simulink model "modelo_naolinear"  (R2018a)
settings: Solver=ode4  StartTime=0.0  StopTime=T_sim  FixedStep=dt  RelTol=1e-3  EnableMultiTasking=on
InitFcn:
  | modelo_naolinear_params
values from neighbouring files (symbols this model uses):
  B22 = B(7:12,2:4)    [main_model2.m]    (also in main_modelo_linear_v1.m; main_modelo_nao_linear_v2.m; modelo_naolinear.m; modelo_naolinear_params.m)
  feed_forward_motor = 2.0    (= 2)    [modelo_naolinear.m]    (also in modelo_naolinear_params.m = 0.5)
  G = inv(K*B22*inv(R)*B22'-A22')*C'*Q    [modelo_naolinear.m]    (also in modelo_naolinear_params.m)
  g = 9.8    [main_model1.m]    (also in main_model2.m; main_modelo_linear_v1.m; main_modelo_linear_v2.m; main_modelo_nao_linear_v1.m)
  incluir_din_motor = -1    [main_model1.m]    (also in main_model2.m; main_modelo_nao_linear_v1.m = 1; main_modelo_nao_linear_v2.m; modelo_naolinear.m = 1)
  Ir = 1e-3    (= 0.001)    [main_model1.m]    (also in main_model2.m; main_modelo_linear_v1.m = 0.01; main_modelo_linear_v2.m = 0.01; main_modelo_nao_linear_v1.m)
  Ixx = 1e-2    (= 0.01)    [main_model1.m]    (also in main_model2.m; main_modelo_linear_v1.m; main_modelo_linear_v2.m; main_modelo_nao_linear_v1.m)
  Iyy = 1e-2    (= 0.01)    [main_model1.m]    (also in main_model2.m; main_modelo_linear_v1.m; main_modelo_linear_v2.m; main_modelo_nao_linear_v1.m)
  Izz = 1.8e-2    (= 0.018)    [main_model1.m]    (also in main_model2.m; main_modelo_linear_v1.m; main_modelo_linear_v2.m; main_modelo_nao_linear_v1.m)
  K = are(A22, B22*inv(R)*B22',C'*Q*C)    [modelo_naolinear.m]    (also in modelo_naolinear_params.m)
  Kd_rot = 0.01    [main_model1.m]    (also in main_model2.m; main_modelo_linear_v1.m = 0; main_modelo_linear_v2.m = 0; main_modelo_nao_linear_v1.m)
  Kd_trans = 0.002    [main_model1.m]    (also in main_model2.m = -0.13723; main_modelo_linear_v1.m = 0; main_modelo_linear_v2.m = 0; main_modelo_nao_linear_v1.m)
  Ki_rot = 1.0    (= 1)    [main_model1.m]    (also in main_model2.m; main_modelo_linear_v1.m = 0.5; main_modelo_linear_v2.m = 0.5; main_modelo_nao_linear_v1.m)
  Ki_trans = 0.06    [main_model1.m]    (also in main_model2.m = 0.41774; main_modelo_linear_v1.m = 0; main_modelo_linear_v2.m = 1; main_modelo_nao_linear_v1.m)
  Kp = 0.9182    [main_model1.m]    (also in main_model2.m; main_modelo_nao_linear_v1.m; main_modelo_nao_linear_v2.m; modelo_naolinear.m)
  Kp_rot = 10    [main_model1.m]    (also in main_model2.m; main_modelo_linear_v1.m = 1; main_modelo_linear_v2.m = 1; main_modelo_nao_linear_v1.m)
  Kp_trans = 0.4    [main_model1.m]    (also in main_model2.m = 2.0968; main_modelo_linear_v1.m = 1; main_modelo_linear_v2.m = 2; main_modelo_nao_linear_v1.m)
  m = 1.0428    [main_model1.m]    (also in main_model2.m; main_modelo_linear_v1.m = 1; main_modelo_linear_v2.m = 1; main_modelo_nao_linear_v1.m)
  N_rot = 100    [main_model2.m]    (also in main_modelo_nao_linear_v2.m; modelo_naolinear.m; modelo_naolinear_params.m)
  N_trans = 5.5815    [main_model2.m]    (also in main_modelo_nao_linear_v2.m; modelo_naolinear.m; modelo_naolinear_params.m)
  p0 = 0    [main_model2.m]    (also in main_modelo_linear_v1.m; main_modelo_linear_v2.m; main_modelo_nao_linear_v2.m; modelo_naolinear.m)
  phi0 = 0    [main_model1.m]    (also in main_model2.m; main_modelo_linear_v1.m; main_modelo_linear_v2.m; main_modelo_nao_linear_v1.m)
  psi0 = 0    [main_model1.m]    (also in main_model2.m; main_modelo_linear_v1.m; main_modelo_linear_v2.m; main_modelo_nao_linear_v1.m)
  q0 = 0    [main_model2.m]    (also in main_modelo_linear_v1.m; main_modelo_linear_v2.m; main_modelo_nao_linear_v2.m; modelo_naolinear.m)
  R = diag([r11,r22,r33])    [main_model2.m]    (also in main_modelo_nao_linear_v2.m; modelo_naolinear.m; modelo_naolinear_params.m)
  r0 = 0    [main_model2.m]    (also in main_modelo_linear_v1.m; main_modelo_linear_v2.m; main_modelo_nao_linear_v2.m; modelo_naolinear.m)
  T = [kf,kf,kf,kf ... (first row only)    [main_model1.m]    (also in main_model2.m; main_modelo_nao_linear_v1.m; main_modelo_nao_linear_v2.m; modelo_naolinear.m)
  T_inv = T^(-1)    [main_model1.m]    (also in main_model2.m; main_modelo_nao_linear_v1.m; main_modelo_nao_linear_v2.m; modelo_naolinear.m)
  tau_a = 0.0569    [main_model1.m]    (also in main_model2.m; main_modelo_nao_linear_v1.m; main_modelo_nao_linear_v2.m; modelo_naolinear.m)
  tau_s = 0.0452    [main_model1.m]    (also in main_model2.m; main_modelo_nao_linear_v1.m; main_modelo_nao_linear_v2.m; modelo_naolinear.m)
  theta0 = 0    [main_model1.m]    (also in main_model2.m; main_modelo_linear_v1.m; main_modelo_linear_v2.m; main_modelo_nao_linear_v1.m)
  vx0 = 0    [main_model1.m]    (also in main_model2.m; main_modelo_nao_linear_v1.m; main_modelo_nao_linear_v2.m; modelo_naolinear.m)
  vy0 = 0    [main_model1.m]    (also in main_model2.m; main_modelo_nao_linear_v1.m; main_modelo_nao_linear_v2.m; modelo_naolinear.m)
  vz0 = 0    [main_model1.m]    (also in main_model2.m; main_modelo_nao_linear_v1.m; main_modelo_nao_linear_v2.m; modelo_naolinear.m)
  x0 = 0    [main_model1.m]    (also in main_model2.m; main_modelo_linear_v1.m; main_modelo_linear_v2.m; main_modelo_nao_linear_v1.m)
  y0 = 0    [main_model1.m]    (also in main_model2.m; main_modelo_linear_v1.m; main_modelo_linear_v2.m; main_modelo_nao_linear_v1.m)
  z0 = 1    [main_model1.m]    (also in main_model2.m; main_modelo_linear_v1.m; main_modelo_linear_v2.m; main_modelo_nao_linear_v1.m)
undefined symbols (not defined in the file or in its folder): sigbuilder_block
libraries: simulink x6
settings Model: Creator=dferr  LastModifiedBy=diego
settings SolverCC: AutoInsertRateTranBlk=on
settings DataIOCC: LimitDataPoints=on  SaveFormat=Array
settings OptimizationCC: LifeSpan=inf
settings DebuggingCC: SFUnexpectedBacktrackingDiag=warning  SFNoUnconditionalDefaultTransitionDiag=warning  SFExecutionAtInitializationDiag=none
settings HardwareCC: ProdBitPerPointer=32  ProdBitPerSizeT=32  ProdBitPerPtrDiffT=32  ProdLargestAtomicFloat=None  ProdIntDivRoundTo=Undefined  ProdEndianess=Unspecified  ProdWordSize=32  ProdHWDeviceType=32-bit Generic
settings ModelReferenceCC: PropagateSignalLabelsOutOfModel=off
settings CodeAppCC: StateflowObjectComments=on
settings GRTTargetCC: TargetLangStandard=C89/C90 (ANSI)  GeneratePreprocessorConditionals=Disable all
settings ConfigComp: CovMetricSettings=dw  CovHtmlReporting=on  CovSaveCumulativeToWorkspaceVar=on  CovSaveSingleToWorkspaceVar=on  CovExternalEMLEnable=off  CovSFcnEnable=off

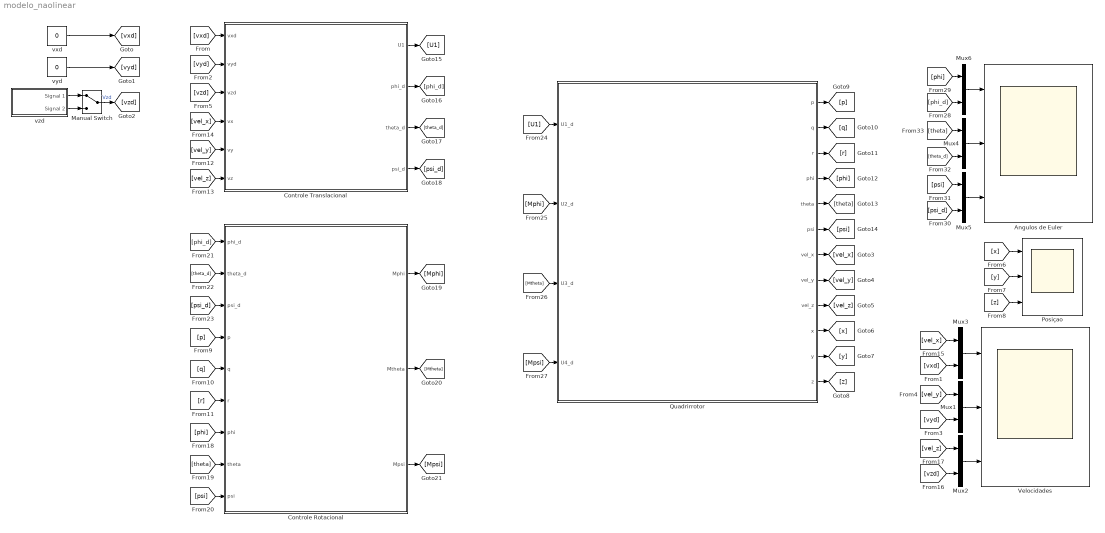
== system modelo_naolinear ==
  Angulos de Euler : Scope  NumInputPorts=3
  Controle Rotacional : Subsystem
      mask Display:
      | disp('Controle Rotacional')
      | port_label('input',1,'phi_d')
      | port_label('input',2,'theta_d')
      | port_label('input',3,'psi_d')
      | port_label('input',4,'p')
      | port_label('input',5,'q')
      | port_label('input',6,'r')
      | port_label('input',7,'phi')
      | port_label('input',8,'theta')
      | port_label('input',9,'psi')
      | port_label('output',1,'Mphi')
      | port_label('output',2,'Mtheta')
      | port_label('output',3,'Mpsi')
  Controle Translacional : Subsystem
      mask Display:
      | disp('Controle Translacional')
      | port_label('input',1,'vxd')
      | port_label('input',2,'vyd')
      | port_label('input',3,'vzd')
      | port_label('input',4,'vx')
      | port_label('input',5,'vy')
      | port_label('input',6,'vz')
      | port_label('output',1,'U1')
      | port_label('output',2,'phi_d')
      | port_label('output',3,'theta_d')
      | port_label('output',4,'psi_d')
  Manual Switch : ManualSwitch
  Mux{1..6} (6 alike) : Mux  Inputs=2
  Posiçao : Scope  NumInputPorts=3
  Quadrirrotor : Subsystem
      mask Display:
      | disp('Quadrirrotor')
      | port_label('input',1,'U1')
      | port_label('input',2,'U2')
      | port_label('input',3,'U3')
      | port_label('input',4,'U4')
      | port_label('output',1,'p')
      | port_label('output',2,'q')
      | port_label('output',3,'r')
      | port_label('output',4,'phi')
      | port_label('output',5,'theta')
      | port_label('output',6,'psi')
      | port_label('output',7,'vel_x')
      | port_label('output',8,'vel_y')
      | port_label('output',9,'vel_z')
      | port_label('output',10,'x')
      | port_label('output',11,'y')
      | port_label('output',12,'z')
  Velocidades : Scope  NumInputPorts=3
  vxd : Constant  Value=0
  vyd : Constant  Value=0
  vzd : Subsystem  Tag=STV Subsys  LoadFcn=sigbuilder_block('load');  StartFcn=sigbuilder_block('start');  StopFcn=sigbuilder_block('stop');  ClipboardFcn=sigbuilder_block('clipboard');  mask(Sigbuilder block){tuvar=[0:10]}
      mask help: Simulink:masks:SigbuilderBlock_MD
      mask init:
      | if ~strcmp(get_param(bdroot(gcbh),'SimulationStatus'),'stopped') tuvar = sigbuilder_block('maskInit'); end
      settings: CopyFcn=sigbuilder_block('copy');  DeleteFcn=sigbuilder_block('delete');  ModelCloseFcn=sigbuilder_block('modelClose');  PreSaveFcn=sigbuilder_block('preSave');  PauseFcn=sigbuilder_block('pause');  ContinueFcn=sigbuilder_block('continue');  NameChangeFcn=sigbuilder_block('namechange');  OpenFcn=sigbuilder_block('open',[437.6 199.2 550.4 400 ]);  CloseFcn=sigbuilder_block('close');
      mask Display: plot(0, 0, 100, 100,[2, 2, 32, 32, 2], [68, 8, 8, 68, 68],[32, 2], [38, 38], [32, 19, 2],[53, 60, 44], [32, 17, 17, 2],[16, 16, 31, 31]);txt = getActiveGroup(gcbh);text(2, 100, txt,'verticalAlignment', 'top');
  wires:
  Mux3/1 -> Velocidades/1
  vzd/1(Signal 1) -> Manual Switch/1
  vzd/2(Signal 2) -> Manual Switch/2
  vxd/1 -> [vxd]
  [vxd] -> Controle Translacional/1(vxd)
  [vxd] -> Mux3/2
  vyd/1 -> [vyd]
  [vyd] -> Controle Translacional/2(vyd)
  Manual Switch/1 -> [vzd]  "Vzd"
  [vzd] -> Controle Translacional/3(vzd)
  [x] -> Posiçao/1
  [y] -> Posiçao/2
  [z] -> Posiçao/3
  [vel_x] -> Controle Translacional/4(vx)
  [vel_y] -> Controle Translacional/5(vy)
  [vel_z] -> Controle Translacional/6(vz)
  [vel_x] -> Mux3/1
  [vel_y] -> Mux1/1
  [vyd] -> Mux1/2
  Mux1/1 -> Velocidades/2
  Mux2/1 -> Velocidades/3
  [vzd] -> Mux2/2
  [vel_z] -> Mux2/1
  Quadrirrotor/7(vel_x) -> [vel_x]
  Quadrirrotor/8(vel_y) -> [vel_y]
  Quadrirrotor/9(vel_z) -> [vel_z]
  Quadrirrotor/10(x) -> [x]
  Quadrirrotor/11(y) -> [y]
  Quadrirrotor/12(z) -> [z]
  Quadrirrotor/1(p) -> [p]
  Quadrirrotor/2(q) -> [q]
  Quadrirrotor/3(r) -> [r]
  Quadrirrotor/4(phi) -> [phi]
  Quadrirrotor/5(theta) -> [theta]
  Quadrirrotor/6(psi) -> [psi]
  [p] -> Controle Rotacional/4(p)
  [q] -> Controle Rotacional/5(q)
  [r] -> Controle Rotacional/6(r)
  [phi] -> Controle Rotacional/7(phi)
  [theta] -> Controle Rotacional/8(theta)
  [psi] -> Controle Rotacional/9(psi)
  Controle Translacional/1(U1) -> [U1]
  Controle Translacional/2(phi_d) -> [phi_d]
  Controle Translacional/3(theta_d) -> [theta_d]
  Controle Translacional/4(psi_d) -> [psi_d]
  [phi_d] -> Controle Rotacional/1(phi_d)
  [theta_d] -> Controle Rotacional/2(theta_d)
  [psi_d] -> Controle Rotacional/3(psi_d)
  [U1] -> Quadrirrotor/1(U1_d)
  Controle Rotacional/1(Mphi) -> [Mphi]
  Controle Rotacional/2(Mtheta) -> [Mtheta]
  Controle Rotacional/3(Mpsi) -> [Mpsi]
  [Mpsi] -> Quadrirrotor/4(U4_d)
  [psi] -> Mux5/1
  [psi_d] -> Mux5/2
  Mux5/1 -> Angulos de Euler/3
  Mux4/1 -> Angulos de Euler/2
  [theta_d] -> Mux4/2
  [theta] -> Mux4/1
  [phi] -> Mux6/1
  [phi_d] -> Mux6/2
  Mux6/1 -> Angulos de Euler/1
  [Mphi] -> Quadrirrotor/2(U2_d)
  [Mtheta] -> Quadrirrotor/3(U3_d)

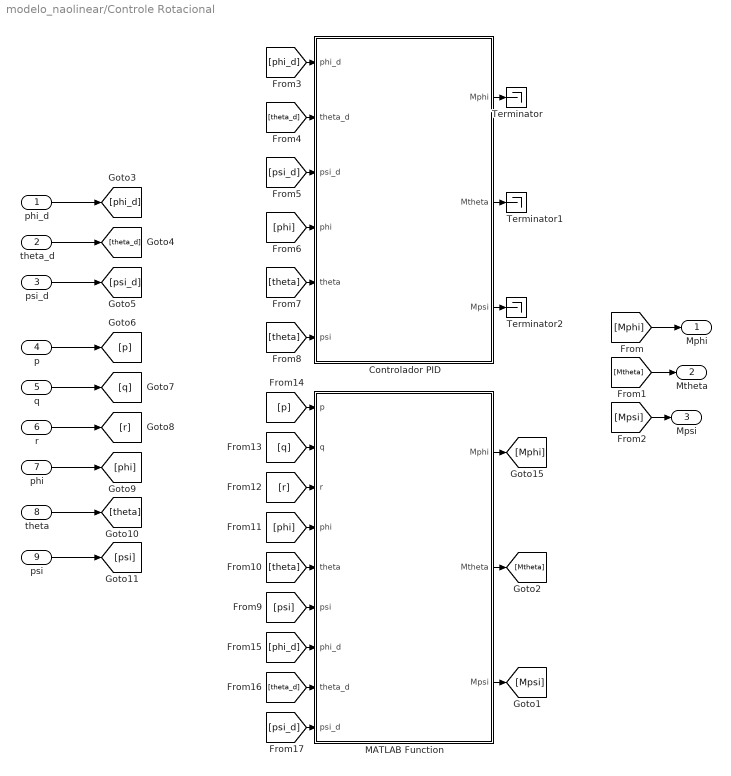
== system modelo_naolinear/Controle Rotacional ==
  phi_d : Inport
  theta_d : Inport  Port=2
  psi_d : Inport  Port=3
  p : Inport  Port=4
  q : Inport  Port=5
  r : Inport  Port=6
  phi : Inport  Port=7
  theta : Inport  Port=8
  psi : Inport  Port=9
  Controlador PID : Subsystem
      mask Display:
      | disp('Controlador PID')
      | port_label('input',1,'phi_d')
      | port_label('input',2,'theta_d')
      | port_label('input',3,'psi_d')
      | port_label('input',4,'phi')
      | port_label('input',5,'theta')
      | port_label('input',6,'psi')
      | port_label('output',1,'Mphi')
      | port_label('output',2,'Mtheta')
      | port_label('output',3,'Mpsi')
  MATLAB Function : MATLAB Function  TreatAsAtomicUnit=on
  Terminator : Terminator
  Terminator1 : Terminator
  Terminator2 : Terminator
  Mphi : Outport
  Mtheta : Outport  Port=2
  Mpsi : Outport  Port=3
  wires:
  [Mphi] -> Mphi/1
  [Mtheta] -> Mtheta/1
  [Mpsi] -> Mpsi/1
  phi_d/1 -> [phi_d]
  theta_d/1 -> [theta_d]
  psi_d/1 -> [psi_d]
  p/1 -> [p]
  q/1 -> [q]
  r/1 -> [r]
  phi/1 -> [phi]
  theta/1 -> [theta]
  psi/1 -> [psi]
  [phi_d] -> Controlador PID/1(phi_d)
  [theta_d] -> Controlador PID/2(theta_d)
  [psi_d] -> Controlador PID/3(psi_d)
  [phi] -> Controlador PID/4(phi)
  [theta] -> Controlador PID/5(theta)
  [theta] -> Controlador PID/6(psi)
  Controlador PID/3(Mpsi) -> Terminator2/1
  Controlador PID/2(Mtheta) -> Terminator1/1
  Controlador PID/1(Mphi) -> Terminator/1
  [psi] -> MATLAB Function/6(psi)
  [theta] -> MATLAB Function/5(theta)
  [phi] -> MATLAB Function/4(phi)
  [r] -> MATLAB Function/3(r)
  [q] -> MATLAB Function/2(q)
  [p] -> MATLAB Function/1(p)
  [phi_d] -> MATLAB Function/7(phi_d)
  [theta_d] -> MATLAB Function/8(theta_d)
  [psi_d] -> MATLAB Function/9(psi_d)
  MATLAB Function/1(Mphi) -> [Mphi]
  MATLAB Function/2(Mtheta) -> [Mtheta]
  MATLAB Function/3(Mpsi) -> [Mpsi]

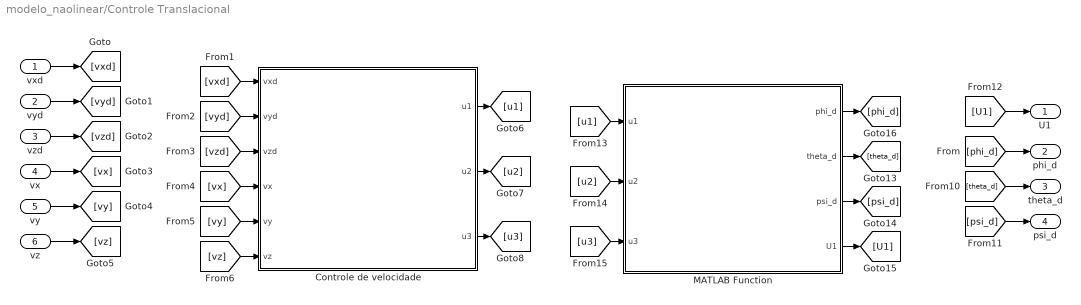
== system modelo_naolinear/Controle Translacional ==
  vxd : Inport
  vyd : Inport  Port=2
  vzd : Inport  Port=3
  vx : Inport  Port=4
  vy : Inport  Port=5
  vz : Inport  Port=6
  Controle de velocidade : Subsystem
      mask Display:
      | disp('Controle de Velocidade PID')
      | port_label('input',1,'vxd')
      | port_label('input',2,'vyd')
      | port_label('input',3,'vzd')
      | port_label('input',4,'vx')
      | port_label('input',5,'vy')
      | port_label('input',6,'vz')
      | 
      | port_label('output',1,'u1')
      | port_label('output',2,'u2')
      | port_label('output',3,'u3')
  MATLAB Function : MATLAB Function  TreatAsAtomicUnit=on
  U1 : Outport
  phi_d : Outport  Port=2
  theta_d : Outport  Port=3
  psi_d : Outport  Port=4
  wires:
  vxd/1 -> [vxd]
  vyd/1 -> [vyd]
  vzd/1 -> [vzd]
  vx/1 -> [vx]
  vy/1 -> [vy]
  vz/1 -> [vz]
  [vxd] -> Controle de velocidade/1(vxd)
  [vyd] -> Controle de velocidade/2(vyd)
  [vzd] -> Controle de velocidade/3(vzd)
  [vx] -> Controle de velocidade/4(vx)
  [vy] -> Controle de velocidade/5("vy ")
  [vz] -> Controle de velocidade/6(vz)
  Controle de velocidade/1(u1) -> [u1]
  Controle de velocidade/2(u2) -> [u2]
  Controle de velocidade/3(u3) -> [u3]
  [phi_d] -> phi_d/1
  [theta_d] -> theta_d/1
  [psi_d] -> psi_d/1
  [U1] -> U1/1
  [u1] -> MATLAB Function/1(u1)
  [u2] -> MATLAB Function/2(u2)
  [u3] -> MATLAB Function/3(u3)
  MATLAB Function/1(phi_d) -> [phi_d]
  MATLAB Function/2(theta_d) -> [theta_d]
  MATLAB Function/3(psi_d) -> [psi_d]
  MATLAB Function/4(U1) -> [U1]

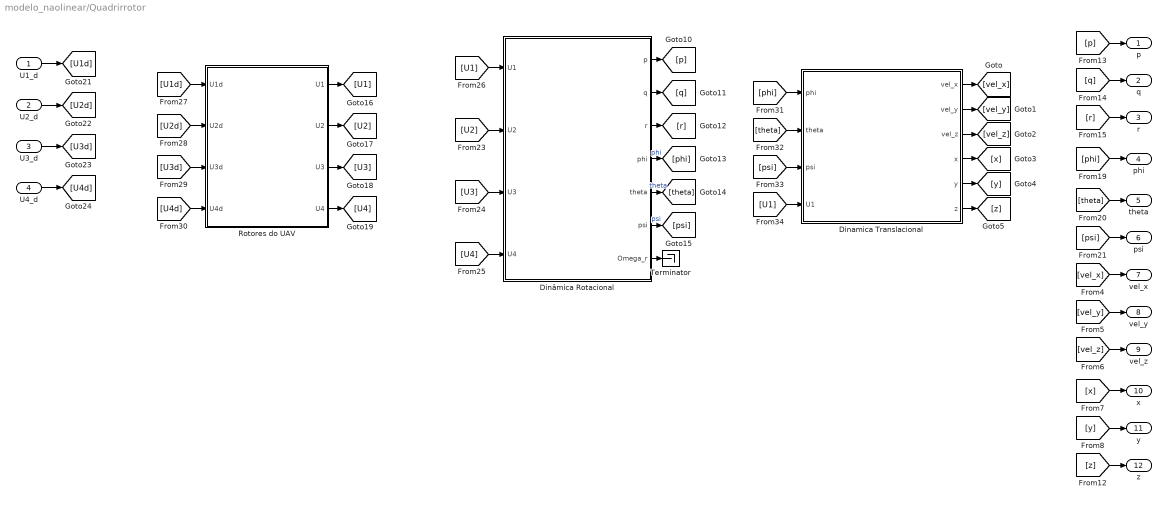
== system modelo_naolinear/Quadrirrotor ==
  U1_d : Inport
  U2_d : Inport  Port=2
  U3_d : Inport  Port=3
  U4_d : Inport  Port=4
  Dinamica Translacional : Subsystem
  Dinâmica Rotacional : Subsystem
      mask Display:
      | disp('Dinâmica Rotacional')
      | port_label('input',1,'U1')
      | port_label('input',2,'U2')
      | port_label('input',3,'U3')
      | port_label('input',4,'U4')
      | port_label('output',1,'p')
      | port_label('output',2,'q')
      | port_label('output',3,'r')
      | port_label('output',4,'phi')
      | port_label('output',5,'theta')
      | port_label('output',6,'psi')
      | port_label('output',7,'Omega_r')
  "Rotores do UAV " : Subsystem
      mask Display:
      | disp('Dinâmica Motores')
      | port_label('input',1,'U1d')
      | port_label('input',2,'U2d')
      | port_label('input',3,'U3d')
      | port_label('input',4,'U4d')
      | port_label('output',1,'U1')
      | port_label('output',2,'U2')
      | port_label('output',3,'U3')
      | port_label('output',4,'U4')
  Terminator : Terminator
  p : Outport
  q : Outport  Port=2
  r : Outport  Port=3
  phi : Outport  Port=4
  theta : Outport  Port=5
  psi : Outport  Port=6
  vel_x : Outport  Port=7
  vel_y : Outport  Port=8
  vel_z : Outport  Port=9
  x : Outport  Port=10
  y : Outport  Port=11
  z : Outport  Port=12
  wires:
  [vel_x] -> vel_x/1
  [vel_y] -> vel_y/1
  [vel_z] -> vel_z/1
  [z] -> z/1
  [y] -> y/1
  [x] -> x/1
  Dinâmica Rotacional/3(r) -> [r]
  Dinâmica Rotacional/2(q) -> [q]
  Dinâmica Rotacional/1(p) -> [p]
  [p] -> p/1
  [q] -> q/1
  [r] -> r/1
  Dinâmica Rotacional/5(theta) -> [theta]  "theta"
  Dinâmica Rotacional/6(psi) -> [psi]  "psi"
  [phi] -> phi/1
  [theta] -> theta/1
  [psi] -> psi/1
  "Rotores do UAV "/1(U1) -> [U1]
  "Rotores do UAV "/2(U2) -> [U2]
  "Rotores do UAV "/3(U3) -> [U3]
  "Rotores do UAV "/4(U4) -> [U4]
  [U1d] -> "Rotores do UAV "/1(U1d)
  [U2d] -> "Rotores do UAV "/2(U2d)
  [U3d] -> "Rotores do UAV "/3(U3d)
  [U4d] -> "Rotores do UAV "/4(U4d)
  U1_d/1 -> [U1d]
  U2_d/1 -> [U2d]
  U3_d/1 -> [U3d]
  U4_d/1 -> [U4d]
  [U4] -> Dinâmica Rotacional/4(U4)
  [U3] -> Dinâmica Rotacional/3(U3)
  [U2] -> Dinâmica Rotacional/2(U2)
  [U1] -> Dinâmica Rotacional/1(U1)
  Dinâmica Rotacional/7(Omega_r) -> Terminator/1
  Dinâmica Rotacional/4(phi) -> [phi]  "phi"
  [phi] -> Dinamica Translacional/1(phi)
  [theta] -> Dinamica Translacional/2(theta)
  [psi] -> Dinamica Translacional/3(psi)
  [U1] -> Dinamica Translacional/4(U1)
  Dinamica Translacional/1(vel_x) -> [vel_x]
  Dinamica Translacional/2(vel_y) -> [vel_y]
  Dinamica Translacional/3(vel_z) -> [vel_z]
  Dinamica Translacional/4(x) -> [x]
  Dinamica Translacional/5(y) -> [y]
  Dinamica Translacional/6(z) -> [z]

== system modelo_naolinear/vzd ==
  Demux : Demux  Tag=STV Demux  Outputs=2
  FromWs : FromWorkspace  Tag=STV FromWs  VariableName=tuvar  SampleTime=0
      SigBuilderData=|
      | common.afterFinalStr = 'Extrapolate'
      | common.sampleTime = 0
      | dataSet.timeRange = [0 20]
      | dataSet.name = 'Group 1'
      | sbobj.Groups.Name = 'Group 1'
      | sbobj.Groups.Signals(1).Name = 'Signal 1'
      | sbobj.Groups.Signals(1).XData = [0 2.05 4.75 8 18 20]
      | sbobj.Groups.Signals(1).YData = [-0.2 8.5 20 20 0 0]
      | sbobj.Groups.Signals(2).Name = 'Signal 2'
      | sbobj.Groups.Signals(2).XData = [0 5 5 20]
      | sbobj.Groups.Signals(2).YData = [0 0 1 1]
      | sbobj.Groups.TimeRange = [0 20]
  Signal 1 : Outport  Tag=STV Outport
  Signal 2 : Outport  Tag=STV Outport  Port=2
  wires:
  FromWs/1 -> Demux/1
  Demux/1 -> Signal 1/1
  Demux/2 -> Signal 2/1

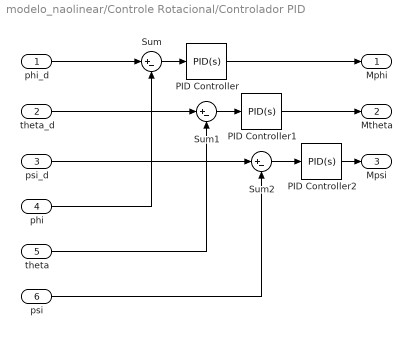
== system modelo_naolinear/Controle Rotacional/Controlador PID ==
  phi_d : Inport
  theta_d : Inport  Port=2
  psi_d : Inport  Port=3
  phi : Inport  Port=4
  theta : Inport  Port=5
  psi : Inport  Port=6
  PID Controller : simulink/Continuous/PID Controller  Controller=PID  TimeDomain=Continuous-time  SampleTime=-1  IntegratorMethod=Forward Euler  FilterMethod=Forward Euler  Form=Ideal  UseFilter=on  ControllerParametersSource=internal  P=Kp_rot  I=Ki_rot  D=Kd_rot  N=N_rot  InitialConditionSource=internal  InitialConditionForIntegrator=0  InitialConditionForFilter=0  ExternalReset=none  LimitOutput=off  UpperSaturationLimit=inf  LowerSaturationLimit=-inf  LinearizeAsGain=on  AntiWindupMode=none  Kb=1  TrackingMode=off  Kt=1  PParamMin=[]  PParamMax=[]  IParamMin=[]  IParamMax=[]  DParamMin=[]  DParamMax=[]  NParamMin=[]  NParamMax=[]  KbParamMin=[]  KbParamMax=[]  KtParamMin=[]  KtParamMax=[]  POutMin=[]  POutMax=[]  IOutMin=[]  IOutMax=[]  DOutMin=[]  DOutMax=[]  NOutMin=[]  NOutMax=[]  KbOutMin=[]  KbOutMax=[]  KtOutMin=[]  KtOutMax=[]  IntegratorOutMin=[]  IntegratorOutMax=[]  FilterOutMin=[]  FilterOutMax=[]  SumOutMin=[]  SumOutMax=[]  SumI1OutMin=[]  SumI1OutMax=[]  SumI2OutMin=[]  SumI2OutMax=[]  SumI3OutMin=[]  SumI3OutMax=[]  SumDOutMin=[]  SumDOutMax=[]  SaturationOutMin=[]  SaturationOutMax=[]  IntegratorContinuousStateAttributes=''  IntegratorStateMustResolveToSignalObject=off  IntegratorRTWStateStorageClass=Auto  FilterContinuousStateAttributes=''  FilterStateMustResolveToSignalObject=off  FilterRTWStateStorageClass=Auto  DifferentiatorICPrevScaledInput=0  DifferentiatorOutMin=[]  DifferentiatorOutMax=[]  InitialConditionSetting=State (most efficient)  FilterDiffOutCoefMin=[]  FilterDiffOutCoefMax=[]  SumDenOutMin=[]  SumDenOutMax=[]  SumNumOutMin=[]  SumNumOutMax=[]  ReciprocalOutMin=[]  ReciprocalOutMax=[]  DivideOutMin=[]  DivideOutMax=[]  TunerSelectOption=Transfer Function Based (PID Tuner App)
  PID Controller1 : simulink/Continuous/PID Controller  Controller=PID  TimeDomain=Continuous-time  SampleTime=-1  IntegratorMethod=Forward Euler  FilterMethod=Forward Euler  Form=Ideal  UseFilter=on  ControllerParametersSource=internal  P=Kp_rot  I=Ki_rot  D=Kd_rot  N=N_rot  InitialConditionSource=internal  InitialConditionForIntegrator=0  InitialConditionForFilter=0  ExternalReset=none  LimitOutput=off  UpperSaturationLimit=inf  LowerSaturationLimit=-inf  LinearizeAsGain=on  AntiWindupMode=none  Kb=1  TrackingMode=off  Kt=1  PParamMin=[]  PParamMax=[]  IParamMin=[]  IParamMax=[]  DParamMin=[]  DParamMax=[]  NParamMin=[]  NParamMax=[]  KbParamMin=[]  KbParamMax=[]  KtParamMin=[]  KtParamMax=[]  POutMin=[]  POutMax=[]  IOutMin=[]  IOutMax=[]  DOutMin=[]  DOutMax=[]  NOutMin=[]  NOutMax=[]  KbOutMin=[]  KbOutMax=[]  KtOutMin=[]  KtOutMax=[]  IntegratorOutMin=[]  IntegratorOutMax=[]  FilterOutMin=[]  FilterOutMax=[]  SumOutMin=[]  SumOutMax=[]  SumI1OutMin=[]  SumI1OutMax=[]  SumI2OutMin=[]  SumI2OutMax=[]  SumI3OutMin=[]  SumI3OutMax=[]  SumDOutMin=[]  SumDOutMax=[]  SaturationOutMin=[]  SaturationOutMax=[]  IntegratorContinuousStateAttributes=''  IntegratorStateMustResolveToSignalObject=off  IntegratorRTWStateStorageClass=Auto  FilterContinuousStateAttributes=''  FilterStateMustResolveToSignalObject=off  FilterRTWStateStorageClass=Auto  DifferentiatorICPrevScaledInput=0  DifferentiatorOutMin=[]  DifferentiatorOutMax=[]  InitialConditionSetting=State (most efficient)  FilterDiffOutCoefMin=[]  FilterDiffOutCoefMax=[]  SumDenOutMin=[]  SumDenOutMax=[]  SumNumOutMin=[]  SumNumOutMax=[]  ReciprocalOutMin=[]  ReciprocalOutMax=[]  DivideOutMin=[]  DivideOutMax=[]  TunerSelectOption=Transfer Function Based (PID Tuner App)
  PID Controller2 : simulink/Continuous/PID Controller  Controller=PID  TimeDomain=Continuous-time  SampleTime=-1  IntegratorMethod=Forward Euler  FilterMethod=Forward Euler  Form=Ideal  UseFilter=on  ControllerParametersSource=internal  P=Kp_rot  I=Ki_rot  D=Kd_rot  N=N_rot  InitialConditionSource=internal  InitialConditionForIntegrator=0  InitialConditionForFilter=0  ExternalReset=none  LimitOutput=off  UpperSaturationLimit=inf  LowerSaturationLimit=-inf  LinearizeAsGain=on  AntiWindupMode=none  Kb=1  TrackingMode=off  Kt=1  PParamMin=[]  PParamMax=[]  IParamMin=[]  IParamMax=[]  DParamMin=[]  DParamMax=[]  NParamMin=[]  NParamMax=[]  KbParamMin=[]  KbParamMax=[]  KtParamMin=[]  KtParamMax=[]  POutMin=[]  POutMax=[]  IOutMin=[]  IOutMax=[]  DOutMin=[]  DOutMax=[]  NOutMin=[]  NOutMax=[]  KbOutMin=[]  KbOutMax=[]  KtOutMin=[]  KtOutMax=[]  IntegratorOutMin=[]  IntegratorOutMax=[]  FilterOutMin=[]  FilterOutMax=[]  SumOutMin=[]  SumOutMax=[]  SumI1OutMin=[]  SumI1OutMax=[]  SumI2OutMin=[]  SumI2OutMax=[]  SumI3OutMin=[]  SumI3OutMax=[]  SumDOutMin=[]  SumDOutMax=[]  SaturationOutMin=[]  SaturationOutMax=[]  IntegratorContinuousStateAttributes=''  IntegratorStateMustResolveToSignalObject=off  IntegratorRTWStateStorageClass=Auto  FilterContinuousStateAttributes=''  FilterStateMustResolveToSignalObject=off  FilterRTWStateStorageClass=Auto  DifferentiatorICPrevScaledInput=0  DifferentiatorOutMin=[]  DifferentiatorOutMax=[]  InitialConditionSetting=State (most efficient)  FilterDiffOutCoefMin=[]  FilterDiffOutCoefMax=[]  SumDenOutMin=[]  SumDenOutMax=[]  SumNumOutMin=[]  SumNumOutMax=[]  ReciprocalOutMin=[]  ReciprocalOutMax=[]  DivideOutMin=[]  DivideOutMax=[]  TunerSelectOption=Transfer Function Based (PID Tuner App)
  Sum : Sum  Inputs=|+-
  Sum1 : Sum  Inputs=|+-
  Sum2 : Sum  Inputs=|+-
  Mphi : Outport
  Mtheta : Outport  Port=2
  Mpsi : Outport  Port=3
  wires:
  PID Controller2/1 -> Mpsi/1
  PID Controller1/1 -> Mtheta/1
  PID Controller/1 -> Mphi/1
  Sum/1 -> PID Controller/1
  Sum1/1 -> PID Controller1/1
  Sum2/1 -> PID Controller2/1
  phi_d/1 -> Sum/1
  theta_d/1 -> Sum1/1
  psi_d/1 -> Sum2/1
  phi/1 -> Sum/2
  theta/1 -> Sum1/2
  psi/1 -> Sum2/2

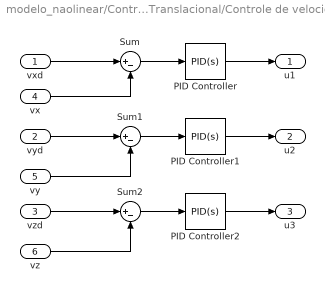
== system modelo_naolinear/Controle Translacional/Controle de velocidade ==
  vxd : Inport
  vyd : Inport  Port=2
  vzd : Inport  Port=3
  vx : Inport  Port=4
  "vy " : Inport  Port=5
  vz : Inport  Port=6
  PID Controller : simulink/Continuous/PID Controller  Controller=PID  TimeDomain=Continuous-time  SampleTime=-1  IntegratorMethod=Forward Euler  FilterMethod=Forward Euler  Form=Parallel  UseFilter=on  ControllerParametersSource=internal  P=Kp_trans  I=Ki_trans  D=Kd_trans  N=N_trans  InitialConditionSource=internal  InitialConditionForIntegrator=0  InitialConditionForFilter=0  ExternalReset=none  LimitOutput=off  UpperSaturationLimit=inf  LowerSaturationLimit=-inf  LinearizeAsGain=on  AntiWindupMode=none  Kb=1  TrackingMode=off  Kt=1  RndMeth=Nearest  PParamMin=[]  PParamMax=[]  IParamMin=[]  IParamMax=[]  DParamMin=[]  DParamMax=[]  NParamMin=[]  NParamMax=[]  KbParamMin=[]  KbParamMax=[]  KtParamMin=[]  KtParamMax=[]  POutMin=[]  POutMax=[]  IOutMin=[]  IOutMax=[]  DOutMin=[]  DOutMax=[]  NOutMin=[]  NOutMax=[]  KbOutMin=[]  KbOutMax=[]  KtOutMin=[]  KtOutMax=[]  IntegratorOutMin=[]  IntegratorOutMax=[]  FilterOutMin=[]  FilterOutMax=[]  SumOutMin=[]  SumOutMax=[]  SumI1OutMin=[]  SumI1OutMax=[]  SumI2OutMin=[]  SumI2OutMax=[]  SumI3OutMin=[]  SumI3OutMax=[]  SumDOutMin=[]  SumDOutMax=[]  SaturationOutMin=[]  SaturationOutMax=[]  IntegratorContinuousStateAttributes=''  IntegratorStateMustResolveToSignalObject=off  IntegratorRTWStateStorageClass=Auto  FilterContinuousStateAttributes=''  FilterStateMustResolveToSignalObject=off  FilterRTWStateStorageClass=Auto  DifferentiatorICPrevScaledInput=0  DifferentiatorOutMin=[]  DifferentiatorOutMax=[]  InitialConditionSetting=State (most efficient)  FilterDiffOutCoefMin=[]  FilterDiffOutCoefMax=[]  SumDenOutMin=[]  SumDenOutMax=[]  SumNumOutMin=[]  SumNumOutMax=[]  ReciprocalOutMin=[]  ReciprocalOutMax=[]  DivideOutMin=[]  DivideOutMax=[]  TunerSelectOption=Transfer Function Based (PID Tuner App)
      settings: LockScale=on
  PID Controller1 : simulink/Continuous/PID Controller  Controller=PID  TimeDomain=Continuous-time  SampleTime=-1  IntegratorMethod=Forward Euler  FilterMethod=Forward Euler  Form=Parallel  UseFilter=on  ControllerParametersSource=internal  P=Kp_trans  I=Ki_trans  D=Kd_trans  N=100  InitialConditionSource=internal  InitialConditionForIntegrator=0  InitialConditionForFilter=0  ExternalReset=none  LimitOutput=off  UpperSaturationLimit=inf  LowerSaturationLimit=-inf  LinearizeAsGain=on  AntiWindupMode=none  Kb=1  TrackingMode=off  Kt=1  RndMeth=Nearest  PParamMin=[]  PParamMax=[]  IParamMin=[]  IParamMax=[]  DParamMin=[]  DParamMax=[]  NParamMin=[]  NParamMax=[]  KbParamMin=[]  KbParamMax=[]  KtParamMin=[]  KtParamMax=[]  POutMin=[]  POutMax=[]  IOutMin=[]  IOutMax=[]  DOutMin=[]  DOutMax=[]  NOutMin=[]  NOutMax=[]  KbOutMin=[]  KbOutMax=[]  KtOutMin=[]  KtOutMax=[]  IntegratorOutMin=[]  IntegratorOutMax=[]  FilterOutMin=[]  FilterOutMax=[]  SumOutMin=[]  SumOutMax=[]  SumI1OutMin=[]  SumI1OutMax=[]  SumI2OutMin=[]  SumI2OutMax=[]  SumI3OutMin=[]  SumI3OutMax=[]  SumDOutMin=[]  SumDOutMax=[]  SaturationOutMin=[]  SaturationOutMax=[]  IntegratorContinuousStateAttributes=''  IntegratorStateMustResolveToSignalObject=off  IntegratorRTWStateStorageClass=Auto  FilterContinuousStateAttributes=''  FilterStateMustResolveToSignalObject=off  FilterRTWStateStorageClass=Auto  DifferentiatorICPrevScaledInput=0  DifferentiatorOutMin=[]  DifferentiatorOutMax=[]  InitialConditionSetting=State (most efficient)  FilterDiffOutCoefMin=[]  FilterDiffOutCoefMax=[]  SumDenOutMin=[]  SumDenOutMax=[]  SumNumOutMin=[]  SumNumOutMax=[]  ReciprocalOutMin=[]  ReciprocalOutMax=[]  DivideOutMin=[]  DivideOutMax=[]  TunerSelectOption=Transfer Function Based (PID Tuner App)
      settings: LockScale=on
  PID Controller2 : simulink/Continuous/PID Controller  Controller=PID  TimeDomain=Continuous-time  SampleTime=-1  IntegratorMethod=Forward Euler  FilterMethod=Forward Euler  Form=Parallel  UseFilter=on  ControllerParametersSource=internal  P=Kp_trans  I=Ki_trans  D=Kd_trans  N=100  InitialConditionSource=internal  InitialConditionForIntegrator=0  InitialConditionForFilter=0  ExternalReset=none  LimitOutput=off  UpperSaturationLimit=inf  LowerSaturationLimit=-inf  LinearizeAsGain=on  AntiWindupMode=none  Kb=1  TrackingMode=off  Kt=1  RndMeth=Nearest  PParamMin=[]  PParamMax=[]  IParamMin=[]  IParamMax=[]  DParamMin=[]  DParamMax=[]  NParamMin=[]  NParamMax=[]  KbParamMin=[]  KbParamMax=[]  KtParamMin=[]  KtParamMax=[]  POutMin=[]  POutMax=[]  IOutMin=[]  IOutMax=[]  DOutMin=[]  DOutMax=[]  NOutMin=[]  NOutMax=[]  KbOutMin=[]  KbOutMax=[]  KtOutMin=[]  KtOutMax=[]  IntegratorOutMin=[]  IntegratorOutMax=[]  FilterOutMin=[]  FilterOutMax=[]  SumOutMin=[]  SumOutMax=[]  SumI1OutMin=[]  SumI1OutMax=[]  SumI2OutMin=[]  SumI2OutMax=[]  SumI3OutMin=[]  SumI3OutMax=[]  SumDOutMin=[]  SumDOutMax=[]  SaturationOutMin=[]  SaturationOutMax=[]  IntegratorContinuousStateAttributes=''  IntegratorStateMustResolveToSignalObject=off  IntegratorRTWStateStorageClass=Auto  FilterContinuousStateAttributes=''  FilterStateMustResolveToSignalObject=off  FilterRTWStateStorageClass=Auto  DifferentiatorICPrevScaledInput=0  DifferentiatorOutMin=[]  DifferentiatorOutMax=[]  InitialConditionSetting=State (most efficient)  FilterDiffOutCoefMin=[]  FilterDiffOutCoefMax=[]  SumDenOutMin=[]  SumDenOutMax=[]  SumNumOutMin=[]  SumNumOutMax=[]  ReciprocalOutMin=[]  ReciprocalOutMax=[]  DivideOutMin=[]  DivideOutMax=[]  TunerSelectOption=Transfer Function Based (PID Tuner App)
      settings: LockScale=on
  Sum : Sum  Inputs=|+-
  Sum1 : Sum  Inputs=|+-
  Sum2 : Sum  Inputs=|+-
  u1 : Outport
  u2 : Outport  Port=2
  u3 : Outport  Port=3
  wires:
  vxd/1 -> Sum/1
  vz/1 -> Sum2/2
  vyd/1 -> Sum1/1
  vzd/1 -> Sum2/1
  vx/1 -> Sum/2
  "vy "/1 -> Sum1/2
  Sum/1 -> PID Controller/1
  PID Controller/1 -> u1/1
  Sum2/1 -> PID Controller2/1
  PID Controller2/1 -> u3/1
  PID Controller1/1 -> u2/1
  Sum1/1 -> PID Controller1/1

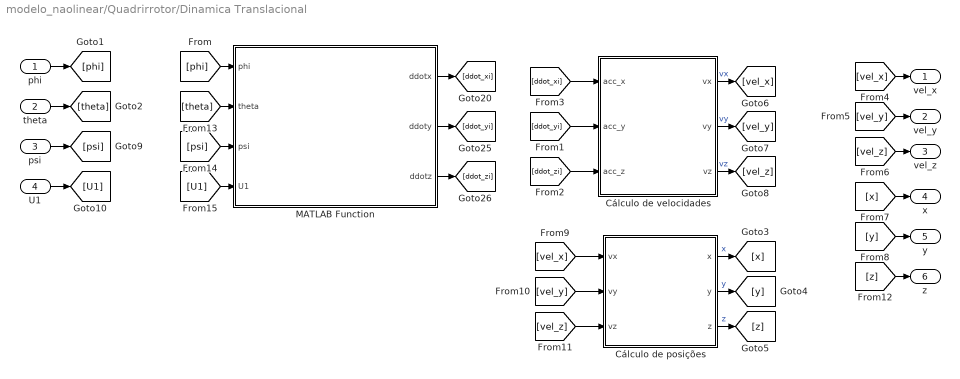
== system modelo_naolinear/Quadrirrotor/Dinamica Translacional ==
  phi : Inport
  theta : Inport  Port=2
  psi : Inport  Port=3
  U1 : Inport  Port=4
  Cálculo de posições : Subsystem
      mask Display:
      | disp('Vel -> Pos')
      | port_label('input',1,'vel_x')
      | port_label('input',2,'vel_y')
      | port_label('input',3,'vel_ z')
      | port_label('output',1,'x')
      | port_label('output',2,'y')
      | port_label('output',3,'z')
  Cálculo de velocidades : Subsystem
      mask Display:
      | disp('Acc -> Vel')
      | port_label('input',1,'acc_x')
      | port_label('input',2,'acc_y')
      | port_label('input',3,'acc_z')
      | port_label('output',1,'vel_x')
      | port_label('output',2,'vel_y')
      | port_label('output',3,'vel_z')
  MATLAB Function : MATLAB Function  TreatAsAtomicUnit=on
  vel_x : Outport
  vel_y : Outport  Port=2
  vel_z : Outport  Port=3
  x : Outport  Port=4
  y : Outport  Port=5
  z : Outport  Port=6
  wires:
  Cálculo de posições/1(x) -> [x]  "x"
  Cálculo de velocidades/3(vz) -> [vel_z]  "vz"
  [ddot_zi] -> Cálculo de velocidades/3(acc_z)
  [ddot_xi] -> Cálculo de velocidades/1(acc_x)
  Cálculo de posições/3(z) -> [z]  "z"
  [ddot_yi] -> Cálculo de velocidades/2(acc_y)
  MATLAB Function/3(ddotz) -> [ddot_zi]
  Cálculo de velocidades/1(vx) -> [vel_x]  "vx"
  Cálculo de posições/2(y) -> [y]  "y"
  MATLAB Function/1(ddotx) -> [ddot_xi]
  [vel_x] -> Cálculo de posições/1(vx)
  MATLAB Function/2(ddoty) -> [ddot_yi]
  Cálculo de velocidades/2(vy) -> [vel_y]  "vy"
  [vel_y] -> Cálculo de posições/2(vy)
  [vel_z] -> Cálculo de posições/3(vz)
  [vel_x] -> vel_x/1
  [vel_y] -> vel_y/1
  [vel_z] -> vel_z/1
  [x] -> x/1
  [y] -> y/1
  [z] -> z/1
  phi/1 -> [phi]
  [phi] -> MATLAB Function/1(phi)
  theta/1 -> [theta]
  [theta] -> MATLAB Function/2(theta)
  psi/1 -> [psi]
  [psi] -> MATLAB Function/3(psi)
  U1/1 -> [U1]
  [U1] -> MATLAB Function/4(U1)

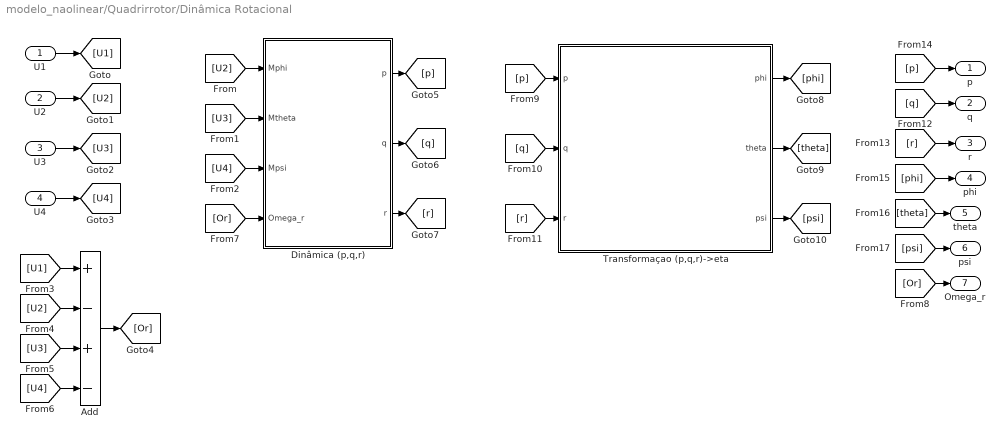
== system modelo_naolinear/Quadrirrotor/Dinâmica Rotacional ==
  U1 : Inport
  U2 : Inport  Port=2
  U3 : Inport  Port=3
  U4 : Inport  Port=4
  Add : Sum  Inputs=+-+-
  Dinâmica (p,q,r) : Subsystem
      mask Display:
      | disp('(p,q,r)')
      | port_label('input',1,'Mphi')
      | port_label('input',2,'Mtheta')
      | port_label('input',3,'Mpsi')
      | port_label('input',4,'Omega_r')
      | port_label('output',1,'p')
      | port_label('output',2,'q')
      | port_label('output',3,'r')
  Transformaçao (p,q,r)->eta : Subsystem  mask(output){}
      mask Display:
      | disp('(p,q,r)-> (phi,theta,psi)')
      | port_label('input',1,'p')
      | port_label('input',2,'q')
      | port_label('input',3,'r')
      | port_label('output',1,'phi')
      | port_label('output',2,'theta')
      | port_label('output',3,'psi')
  p : Outport
  q : Outport  Port=2
  r : Outport  Port=3
  phi : Outport  Port=4
  theta : Outport  Port=5
  psi : Outport  Port=6
  Omega_r : Outport  Port=7
  wires:
  U1/1 -> [U1]
  U2/1 -> [U2]
  U3/1 -> [U3]
  U4/1 -> [U4]
  [U2] -> Dinâmica (p,q,r)/1(Mphi)
  [U3] -> Dinâmica (p,q,r)/2(Mtheta)
  [U4] -> Dinâmica (p,q,r)/3(Mpsi)
  [U1] -> Add/1
  [U2] -> Add/2
  [U3] -> Add/3
  [U4] -> Add/4
  Add/1 -> [Or]
  [Or] -> Dinâmica (p,q,r)/4(Omega_r)
  [Or] -> Omega_r/1
  Dinâmica (p,q,r)/1(p) -> [p]
  Dinâmica (p,q,r)/2(q) -> [q]
  Dinâmica (p,q,r)/3(r) -> [r]
  [p] -> Transformaçao (p,q,r)->eta/1(p)
  [q] -> Transformaçao (p,q,r)->eta/2(q)
  [r] -> Transformaçao (p,q,r)->eta/3(r)
  [p] -> p/1
  [q] -> q/1
  [r] -> r/1
  Transformaçao (p,q,r)->eta/1(phi) -> [phi]
  Transformaçao (p,q,r)->eta/2(theta) -> [theta]
  Transformaçao (p,q,r)->eta/3(psi) -> [psi]
  [phi] -> phi/1
  [theta] -> theta/1
  [psi] -> psi/1

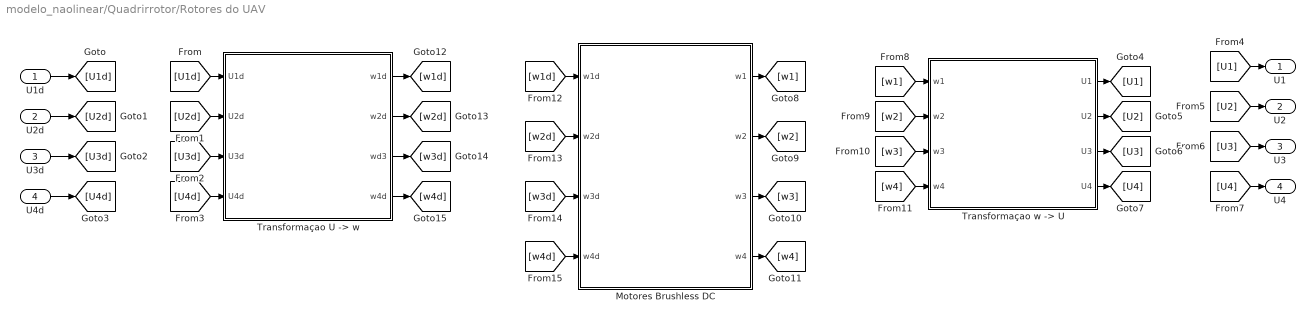
== system modelo_naolinear/Quadrirrotor/Rotores do UAV  ==
  U1d : Inport
  U2d : Inport  Port=2
  U3d : Inport  Port=3
  U4d : Inport  Port=4
  "Motores Brushless DC " : Subsystem
  "Transformaçao U -> w" : Subsystem
  "Transformaçao w -> U" : Subsystem
  U1 : Outport
  U2 : Outport  Port=2
  U3 : Outport  Port=3
  U4 : Outport  Port=4
  wires:
  U2d/1 -> [U2d]
  U3d/1 -> [U3d]
  U4d/1 -> [U4d]
  [U1d] -> "Transformaçao U -> w"/1(U1d)
  [U2d] -> "Transformaçao U -> w"/2(U2d)
  [U3d] -> "Transformaçao U -> w"/3(U3d)
  [U4d] -> "Transformaçao U -> w"/4(U4d)
  [U1] -> U1/1
  [U2] -> U2/1
  [U3] -> U3/1
  [U4] -> U4/1
  "Transformaçao w -> U"/1(U1) -> [U1]
  "Transformaçao w -> U"/2(U2) -> [U2]
  "Transformaçao w -> U"/3(U3) -> [U3]
  "Transformaçao w -> U"/4(U4) -> [U4]
  [w1] -> "Transformaçao w -> U"/1(w1)
  [w2] -> "Transformaçao w -> U"/2(w2)
  [w3] -> "Transformaçao w -> U"/3(w3)
  [w4] -> "Transformaçao w -> U"/4(w4)
  "Transformaçao U -> w"/1(w1d) -> [w1d]
  "Transformaçao U -> w"/2(w2d) -> [w2d]
  "Transformaçao U -> w"/3(wd3) -> [w3d]
  "Transformaçao U -> w"/4(w4d) -> [w4d]
  [w1d] -> "Motores Brushless DC "/1(w1d)
  [w2d] -> "Motores Brushless DC "/2(w2d)
  [w3d] -> "Motores Brushless DC "/3(w3d)
  [w4d] -> "Motores Brushless DC "/4(w4d)
  "Motores Brushless DC "/1(w1) -> [w1]
  "Motores Brushless DC "/2(w2) -> [w2]
  "Motores Brushless DC "/3(w3) -> [w3]
  "Motores Brushless DC "/4(w4) -> [w4]
  U1d/1 -> [U1d]

== system modelo_naolinear/Quadrirrotor/Dinamica Translacional/Cálculo de posições ==
  vx : Inport
  vy : Inport  Port=2
  vz : Inport  Port=3
  Integrator : Integrator  InitialCondition=x0
  Integrator1 : Integrator  InitialCondition=y0
  Integrator2 : Integrator  InitialCondition=z0  LimitOutput=on  LowerSaturationLimit=0
  x : Outport
  y : Outport  Port=2
  z : Outport  Port=3
  wires:
  Integrator/1 -> x/1
  Integrator1/1 -> y/1
  vy/1 -> Integrator1/1
  vz/1 -> Integrator2/1
  vx/1 -> Integrator/1
  Integrator2/1 -> z/1

== system modelo_naolinear/Quadrirrotor/Dinamica Translacional/Cálculo de velocidades ==
  acc_x : Inport
  acc_y : Inport  Port=2
  acc_z : Inport  Port=3
  Integrator : Integrator  InitialCondition=vx0  ZeroCross=off
  Integrator1 : Integrator  InitialCondition=vy0  ZeroCross=off
  Integrator2 : Integrator  InitialCondition=vz0  ZeroCross=off
  vx : Outport
  vy : Outport  Port=2
  vz : Outport  Port=3
  wires:
  Integrator2/1 -> vz/1
  acc_z/1 -> Integrator2/1
  Integrator/1 -> vx/1
  acc_x/1 -> Integrator/1
  acc_y/1 -> Integrator1/1
  Integrator1/1 -> vy/1

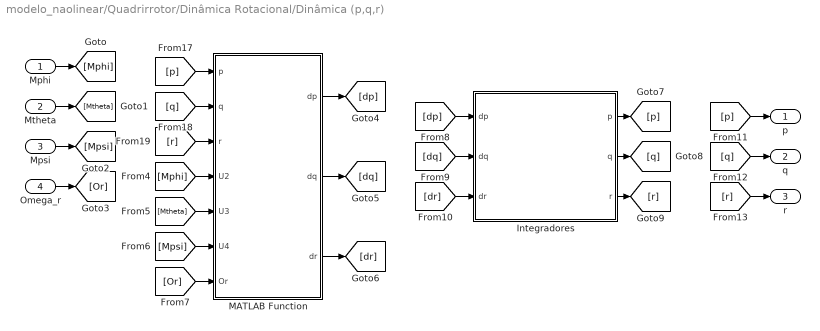
== system modelo_naolinear/Quadrirrotor/Dinâmica Rotacional/Dinâmica (p,q,r) ==
  Mphi : Inport
  Mtheta : Inport  Port=2
  Mpsi : Inport  Port=3
  Omega_r : Inport  Port=4
  Integradores : Subsystem
  MATLAB Function : MATLAB Function  TreatAsAtomicUnit=on
  p : Outport
  q : Outport  Port=2
  r : Outport  Port=3
  wires:
  Mphi/1 -> [Mphi]
  Mtheta/1 -> [Mtheta]
  Mpsi/1 -> [Mpsi]
  Omega_r/1 -> [Or]
  [Or] -> MATLAB Function/7(Or)
  [Mpsi] -> MATLAB Function/6(U4)
  [Mtheta] -> MATLAB Function/5(U3)
  [Mphi] -> MATLAB Function/4(U2)
  MATLAB Function/1(dp) -> [dp]
  MATLAB Function/2(dq) -> [dq]
  [p] -> p/1
  [q] -> q/1
  [r] -> r/1
  [p] -> MATLAB Function/1(p)
  [q] -> MATLAB Function/2(q)
  [r] -> MATLAB Function/3(r)
  MATLAB Function/3(dr) -> [dr]
  [dp] -> Integradores/1(dp)
  [dq] -> Integradores/2(dq)
  [dr] -> Integradores/3(dr)
  Integradores/1(p) -> [p]
  Integradores/2(q) -> [q]
  Integradores/3(r) -> [r]

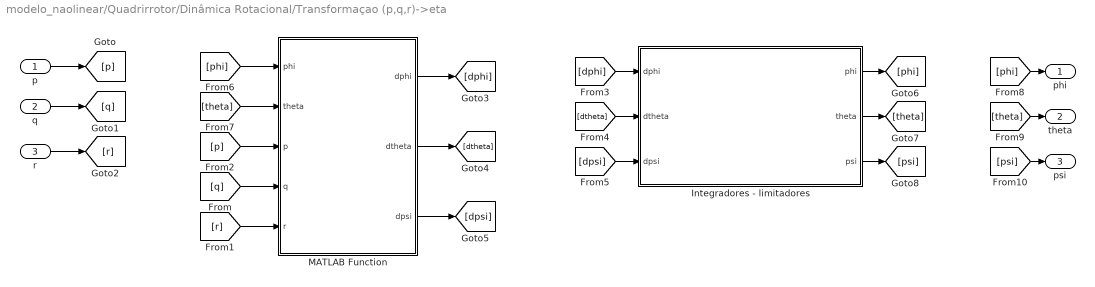
== system modelo_naolinear/Quadrirrotor/Dinâmica Rotacional/Transformaçao (p,q,r)->eta ==
  p : Inport
  q : Inport  Port=2
  r : Inport  Port=3
  Integradores - limitadores : Subsystem
  MATLAB Function : MATLAB Function  TreatAsAtomicUnit=on
  phi : Outport
  theta : Outport  Port=2
  psi : Outport  Port=3
  wires:
  p/1 -> [p]
  q/1 -> [q]
  r/1 -> [r]
  [q] -> MATLAB Function/4(q)
  [r] -> MATLAB Function/5(r)
  [p] -> MATLAB Function/3(p)
  MATLAB Function/1(dphi) -> [dphi]
  MATLAB Function/2(dtheta) -> [dtheta]
  MATLAB Function/3(dpsi) -> [dpsi]
  [phi] -> MATLAB Function/1(phi)
  [theta] -> MATLAB Function/2(theta)
  [phi] -> phi/1
  [theta] -> theta/1
  [psi] -> psi/1
  [dphi] -> Integradores - limitadores/1(dphi)
  [dtheta] -> Integradores - limitadores/2(dtheta)
  [dpsi] -> Integradores - limitadores/3(dpsi)
  Integradores - limitadores/1(phi) -> [phi]
  Integradores - limitadores/2(theta) -> [theta]
  Integradores - limitadores/3(psi) -> [psi]

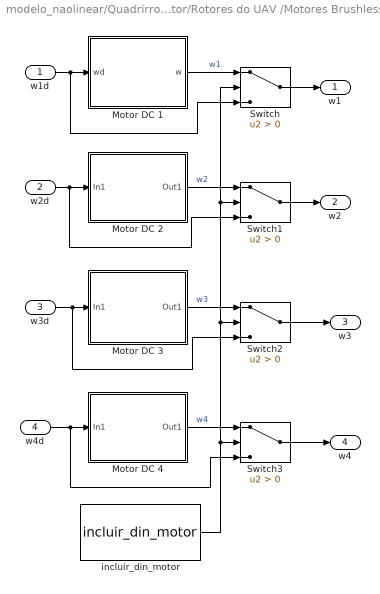
== system modelo_naolinear/Quadrirrotor/Rotores do UAV /Motores Brushless DC  ==
  w1d : Inport
  w2d : Inport  Port=2
  w3d : Inport  Port=3
  w4d : Inport  Port=4
  Motor DC 1 : Subsystem
      mask Display:
      | disp('Motor DC')
      | port_label('input',1,'wd')
      | port_label('output',1,'w')
  Motor DC 2 : Subsystem
      mask Display:
      | disp('Motor DC')
      | port_label('input',1,'wd')
      | port_label('output',1,'w')
  Motor DC 3 : Subsystem
      mask Display:
      | disp('Motor DC')
      | port_label('input',1,'wd')
      | port_label('output',1,'w')
  Motor DC 4 : Subsystem
      mask Display:
      | disp('Motor DC')
      | port_label('input',1,'wd')
      | port_label('output',1,'w')
  Switch{,1..3} (4 alike) : Switch  Criteria=u2 > Threshold
  incluir_din_motor : Constant  Value=incluir_din_motor
  w1 : Outport
  w2 : Outport  Port=2
  w3 : Outport  Port=3
  w4 : Outport  Port=4
  wires:
  Motor DC 4/1(Out1) -> Switch3/1  "w4"
  Switch2/1 -> w3/1
  w4d/1 -> Switch3/3, Motor DC 4/1(In1)
  incluir_din_motor/1 -> Switch/2, Switch1/2, Switch2/2, Switch3/2
  Motor DC 2/1(Out1) -> Switch1/1  "w2"
  Motor DC 1/1(w) -> Switch/1  "w1"
  Motor DC 3/1(Out1) -> Switch2/1  "w3"
  w3d/1 -> Switch2/3, Motor DC 3/1(In1)
  w2d/1 -> Switch1/3, Motor DC 2/1(In1)
  Switch3/1 -> w4/1
  w1d/1 -> Switch/3, Motor DC 1/1(wd)
  Switch/1 -> w1/1
  Switch1/1 -> w2/1

== system modelo_naolinear/Quadrirrotor/Rotores do UAV /Transformaçao U -> w ==
  U1d : Inport
  U2d : Inport  Port=2
  U3d : Inport  Port=3
  U4d : Inport  Port=4
  Bus Creator1 : BusCreator  Inputs=4
  Demux1 : Demux
  Transformação Omega = T^(-1)*U : Gain  Gain=T_inv  Multiplication=Matrix(K*u)  RndMeth=Nearest  LockScale=on
  w1d : Outport
  w2d : Outport  Port=2
  wd3 : Outport  Port=3
  w4d : Outport  Port=4
  wires:
  Bus Creator1/1 -> Transformação Omega = T^(-1)*U/1
  Transformação Omega = T^(-1)*U/1 -> Demux1/1  "Frequências angulares desejadas"
  U3d/1 -> Bus Creator1/3
  U2d/1 -> Bus Creator1/2
  U1d/1 -> Bus Creator1/1
  Demux1/2 -> w2d/1  "w2d"
  U4d/1 -> Bus Creator1/4
  Demux1/3 -> wd3/1  "wd3"
  Demux1/4 -> w4d/1  "w4d"
  Demux1/1 -> w1d/1  "w1d"

== system modelo_naolinear/Quadrirrotor/Rotores do UAV /Transformaçao w -> U ==
  w1 : Inport
  w2 : Inport  Port=2
  w3 : Inport  Port=3
  w4 : Inport  Port=4
  Bus Creator2 : BusCreator  Inputs=4
  Demux : Demux
  Transformação U = T*Omega : Gain  Gain=T  Multiplication=Matrix(K*u)  RndMeth=Nearest  LockScale=on
  U1 : Outport
  U2 : Outport  Port=2
  U3 : Outport  Port=3
  U4 : Outport  Port=4
  wires:
  Bus Creator2/1 -> Transformação U = T*Omega/1
  Transformação U = T*Omega/1 -> Demux/1
  Demux/3 -> U3/1  "U3"
  w4/1 -> Bus Creator2/4
  w1/1 -> Bus Creator2/1
  Demux/2 -> U2/1  "U2"
  w2/1 -> Bus Creator2/2
  w3/1 -> Bus Creator2/3
  Demux/1 -> U1/1  "U1"
  Demux/4 -> U4/1  "U4"

== system modelo_naolinear/Quadrirrotor/Dinâmica Rotacional/Dinâmica (p,q,r)/Integradores ==
  dp : Inport
  dq : Inport  Port=2
  dr : Inport  Port=3
  Integrator3 : Integrator  InitialCondition=p0
  Integrator4 : Integrator  InitialCondition=q0
  Integrator5 : Integrator  InitialCondition=r0
  p : Outport
  q : Outport  Port=2
  r : Outport  Port=3
  wires:
  Integrator3/1 -> p/1
  Integrator4/1 -> q/1
  dp/1 -> Integrator3/1
  dr/1 -> Integrator5/1
  dq/1 -> Integrator4/1
  Integrator5/1 -> r/1

== system modelo_naolinear/Quadrirrotor/Dinâmica Rotacional/Transformaçao (p,q,r)->eta/Integradores - limitadores ==
  dphi : Inport
  dtheta : Inport  Port=2
  dpsi : Inport  Port=3
  -pi<=u<=pi : Fcn  Expr=u - 2*pi*floor( (u+pi)/(2*pi) )
  -pi<=u<=pi1 : Fcn  Expr=u - 2*pi*floor( (u+pi)/(2*pi) )
  -pi<=u<=pi2 : Fcn  Expr=u - 2*pi*floor( (u+pi)/(2*pi) )
  Integrator : Integrator  InitialCondition=phi0
  Integrator1 : Integrator  InitialCondition=theta0
  Integrator2 : Integrator  InitialCondition=psi0
  phi : Outport
  theta : Outport  Port=2
  psi : Outport  Port=3
  wires:
  Integrator/1 -> -pi<=u<=pi/1
  dpsi/1 -> Integrator2/1
  -pi<=u<=pi/1 -> phi/1
  Integrator1/1 -> -pi<=u<=pi1/1
  Integrator2/1 -> -pi<=u<=pi2/1
  -pi<=u<=pi2/1 -> psi/1
  -pi<=u<=pi1/1 -> theta/1
  dphi/1 -> Integrator/1
  dtheta/1 -> Integrator1/1

== system modelo_naolinear/Quadrirrotor/Rotores do UAV /Motores Brushless DC /Motor DC 1 ==
  wd : Inport
  Gain : Gain  Gain=feed_forward_motor
  Modelo Motor 1 : TransferFcn  Numerator=[Kp]  Denominator=[tau_a 1]
  Sum : Sum  Inputs=++|
  Transport Delay : TransportDelay  DelayTime=tau_s
  w : Outport
  wires:
  Sum/1 -> w/1
  Gain/1 -> Sum/1
  Transport Delay/1 -> Modelo Motor 1/1
  Modelo Motor 1/1 -> Sum/2
  wd/1 -> Transport Delay/1, Gain/1

== system modelo_naolinear/Quadrirrotor/Rotores do UAV /Motores Brushless DC /Motor DC 2 ==
  In1 : Inport
  Gain : Gain  Gain=feed_forward_motor
  Modelo Motor 2 : TransferFcn  Numerator=[Kp]  Denominator=[tau_a 1]
  Sum : Sum  Inputs=++|
  Transport Delay : TransportDelay  DelayTime=tau_s
  Out1 : Outport
  wires:
  Gain/1 -> Sum/1
  Sum/1 -> Out1/1  "w2"
  Transport Delay/1 -> Modelo Motor 2/1
  Modelo Motor 2/1 -> Sum/2
  In1/1 -> Transport Delay/1, Gain/1

== system modelo_naolinear/Quadrirrotor/Rotores do UAV /Motores Brushless DC /Motor DC 3 ==
  In1 : Inport
  Gain : Gain  Gain=feed_forward_motor
  Modelo Motor 3 : TransferFcn  Numerator=[Kp]  Denominator=[tau_a 1]
  Sum : Sum  Inputs=++|
  Transport Delay : TransportDelay  DelayTime=tau_s
  Out1 : Outport
  wires:
  Gain/1 -> Sum/1
  Sum/1 -> Out1/1  "w3"
  Transport Delay/1 -> Modelo Motor 3/1
  Modelo Motor 3/1 -> Sum/2
  In1/1 -> Transport Delay/1, Gain/1

== system modelo_naolinear/Quadrirrotor/Rotores do UAV /Motores Brushless DC /Motor DC 4 ==
  In1 : Inport
  Gain : Gain  Gain=feed_forward_motor
  Modelo Motor 4 : TransferFcn  Numerator=[Kp]  Denominator=[tau_a 1]
  Sum : Sum  Inputs=++|
  Transport Delay : TransportDelay  DelayTime=tau_s
  Out1 : Outport
  wires:
  Gain/1 -> Sum/1
  Sum/1 -> Out1/1  "w4"
  Transport Delay/1 -> Modelo Motor 4/1
  Modelo Motor 4/1 -> Sum/2
  In1/1 -> Transport Delay/1, Gain/1

== matlab function modelo_naolinear/Quadrirrotor/Dinâmica Rotacional/Transformaçao (p,q,r)->eta/MATLAB Function ==
  data: phi input; dphi output; theta input; p input; q input; r input; dtheta output; dpsi output
function [dphi, dtheta, dpsi] = pqr_eta_rhs(phi, theta,p,q,r)

dphi = (r*cos(phi) + q*sin(phi))*tan(theta) + p;
dtheta = q*cos(phi) - r*sin(phi);
dpsi = (cos(phi)/cos(theta))*r + (sin(phi)/cos(theta))*q;
end

== matlab function modelo_naolinear/Quadrirrotor/Dinâmica Rotacional/Dinâmica (p,q,r)/MATLAB Function ==
  data: p input; q input; dp output size=1; r input; U2 input; U3 input; U4 input; Or input; dq output size=1; dr output size=1; Ixx parameter; Iyy parameter; Izz parameter; Ir parameter
function [dp, dq, dr] = pqr_rhs(p,q,r,U2,U3,U4,Or, Ixx, Iyy, Izz, Ir)

dp = (Iyy-Izz)*q*r/Ixx - (Ir*Or)*q/Ixx + U2/Ixx;
dq = (Izz-Ixx)*p*r/Iyy - (Ir*Or)*p/Iyy + U3/Iyy;
dr = (Ixx-Iyy)*p*q/Izz + U4/Izz;
end

== matlab function modelo_naolinear/Quadrirrotor/Dinamica Translacional/MATLAB Function ==
  data: phi input; ddotx output; theta input; psi input; U1 input; ddoty output; ddotz output; m parameter; g parameter
function [ddotx, ddoty, ddotz] = din_trans_rhs(phi, theta, psi, U1, m, g)

ddotx = (cos(phi)*cos(psi)*sin(theta) + sin(phi)*sin(psi))*U1/m;
ddoty = (cos(phi)*sin(psi)*sin(theta) - sin(phi)*cos(psi))*U1/m;
ddotz = -g + cos(phi)*cos(theta)*U1/m;
end

== matlab function modelo_naolinear/Controle Translacional/MATLAB Function ==
  data: u1 input; phi_d output; u2 input; u3 input; theta_d output; psi_d output; U1 output; g parameter; m parameter
function [phi_d, theta_d, psi_d, U1] = entradas_virtuais(u1, u2, u3, g, m)
phi_d = atan(-u2/sqrt(u1^2+(g+u3)^2));
theta_d = atan(u1/(g+u3));
psi_d = 0;
U1 = m*sqrt(u1^2 + u2^2 + (g+u3)^2);
end

== matlab function modelo_naolinear/Controle Rotacional/MATLAB Function ==
  data: p input; Mphi output; q input; r input; phi input; theta input; psi input; phi_d input; theta_d input; psi_d input; Mtheta output; Mpsi output; K parameter; G parameter; R parameter; B22 parameter
function [Mphi, Mtheta, Mpsi] = controlador_lqt(p,q,r,...
    phi,theta,psi,phi_d,theta_d,psi_d, K, G, R, B22)
% controlador Lineqr Quadratic Tranking para a dinâmica rotacional.
% assume-se uma dinâmica linear do tipo: 
%
%                    dx/dt = Ax + Bu
%                        y = Dx
% onde:
%   A é uma matriz 6x6
%   B é uma matriz 6x3
%   C é uma matriz 3x6
%
% note que na saída são observados apenas os ângulos de Euler.
%
% O índice de desempenho é:
%
%       J = (1/2)e'He + (1/2)int_{t_0}^{t_f}(e'Qe + u'Ru)dt
%
% onde:
%   e(t) = z(t) - Cx(t), é o erro a ser minimizado
%   z(t) é a referência a ser seguida.
%   As matrizes H, Q e R são de dimensões apropriadas
%
% O controle ótimo é:
%                
%                      u = R^(-1)*B'*(g - Kx)
% onde:
%   g(t) é a solução algébrica da equação:
%
%                0 = (KBR^(-1)B'-A')g - C'Qz
% ou g = Gz, onde
%                G = (KBR^(-1)B'-A')^(-1)C'Q
%
% A matriz K é a solução da ARE
%
%               A'*K + K*A - K*S*K + V = 0
% onde:
%   S = BR^(-1)B'
%   V = C'QC
% -------------------------------------------------------------------------
x = [p;q;r;phi;theta;psi];
z = [phi_d;theta_d;psi_d];
%
g = G*z;
u = inv(R)*B22'*(g-K*x);
Mphi = u(1);
Mtheta = u(2);
Mpsi = u(3);
end
